simulink model "statefeedback"  (R2020a)
settings: Solver=VariableStepAuto  StartTime=0.0  StopTime=10.0  RelTol=1e-3
values from neighbouring files (symbols this model uses):
  K1 = Kba*T    [state_feedback.m]
undefined symbols (not defined in the file or in its folder): A, B, C
settings Model: Creator=wyton  LastModifiedBy=wyton

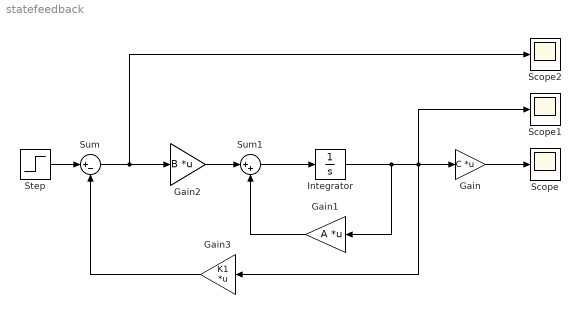
== system statefeedback ==
  Gain : Gain  Gain=C  Multiplication=Matrix(K*u)
      settings: AttributesFormatString=C
  Gain1 : Gain  Gain=A  Multiplication=Matrix(K*u)
      settings: AttributesFormatString=A
  Gain2 : Gain  Tag=B  Gain=B  Multiplication=Matrix(K*u)
      settings: AttributesFormatString=B
  Gain3 : Gain  Gain=K1  Multiplication=Matrix(K*u)
      settings: AttributesFormatString=K
  Integrator : Integrator
  Scope : Scope
      settings: AttributesFormatString=output
  Scope1 : Scope
      settings: AttributesFormatString=state
  Scope2 : Scope
      settings: AttributesFormatString=control
  Step : Step  After=0  SampleTime=0
  Sum : Sum  Inputs=|+-
  Sum1 : Sum  Inputs=|++
  wires:
  Step/1 -> Sum/1
  Sum/1 -> Scope2/1, Gain2/1
  Sum1/1 -> Integrator/1
  Gain2/1 -> Sum1/1
  Integrator/1 -> Gain1/1, Gain3/1, Gain/1, Scope1/1
  Gain1/1 -> Sum1/2
  Gain/1 -> Scope/1
  Gain3/1 -> Sum/2
